simulink model "JSimResultsModel2"  (R2021a)
settings: Solver=VariableStepAuto  StartTime=0.0  StopTime=25  RelTol=1e-3
values from neighbouring files (symbols this model uses):
  A = obj.networkMatrices.A    [Network.m]    (also in Subsystem.m = obj.A{obj.index}; jPaperData1.mat = [7.21225729966 1.39049686205 0 0 -0.282509513675 -0.19440187; jPaperData2.mat = [1.59283418225 -1.98990334273 -0.0774022354425 0.03883188575; paperData.mat = [-0.897343897753 -1.03363634124 0 0 0 0 -1.03363634124 -1.19)
  AcDiss =     [jPaperData1.mat]    (also in jPaperData2.mat)
  AcStab =     [jPaperData1.mat]    (also in jPaperData2.mat = [-4.66639923531 0.0224905641012 0.183856829633 -0.0600919958)
  B = obj.networkMatrices.B    [Network.m]    (also in Subsystem.m = obj.B{obj.index}; jPaperData1.mat = [0.133289291835 -2.25582289472 0 0 0 0 0 0 0 0 0 0 ... (50 e; jPaperData2.mat = [0.884783010265 -0.0578061269532 0 0 0 0 0 0 0 0 0 0 ... (50; paperData.mat = [-0.767652209467 0.0479827696564 0 0 0 0 0 0 0 0.69770450426)
  BcDiss =     [jPaperData1.mat]    (also in jPaperData2.mat)
  BcStab =     [jPaperData1.mat]    (also in jPaperData2.mat = [4.69331758427 -3.97574466957 -0.18243601768 0.0596281142245)
  C = obj.networkMatrices.C    [Network.m]    (also in Subsystem.m = {}; jPaperData1.mat = [-0.398868811937 0 0 0 0 0.199769403633 0 0 0 0 0 0 ... (50 ; jPaperData2.mat = [-2.29277321488 0 0 0 0 1.99520966434 0 0 0 0 0 0.4731154890; paperData.mat = [-0.192732954692 0 0 0.794595441386 0 0 0 1.44304729411 0 0 )
  CcDiss =     [jPaperData1.mat]    (also in jPaperData2.mat)
  CcStab =     [jPaperData1.mat]    (also in jPaperData2.mat = [3.40584102634 0.0670370876354 0 -0.466213574125 0.023320064)
  D = obj.networkMatrices.D    [Network.m]    (also in Subsystem.m = {}; jPaperData1.mat = [0 0 0 0 0 0 0 0 0 0 0 0 ... (25 elements, 5x5)]; jPaperData2.mat = [0 0 0 0 0 0 0 0 0 0 0 0 ... (25 elements, 5x5)]; paperData.mat = [0  0  0; 0  0  0; 0  0  0])
  DcDiss =     [jPaperData1.mat]    (also in jPaperData2.mat)
  DcStab =     [jPaperData1.mat]    (also in jPaperData2.mat = [-0.559949680356 -0.0227155093389 0 0.0369895329508 0.048553)
  E = obj.networkMatrices.E    [Network.m]    (also in Subsystem.m = {}; jPaperData1.mat = [0.013736298283 0.0126277412194 0 0 0 -0.00335268402912 0 0.; jPaperData2.mat = [-0.000849733283809 -0.00431479261265 0.00356522747973 0.001; paperData.mat = [0 0.622727541957 0 0 0 0 -0.10315996141 -0.125734072536 0 -)
  F = obj.networkMatrices.F    [Network.m]    (also in Subsystem.m = {}; jPaperData1.mat = [0 0 0 0 0 0 0.00667542601126 0 0 0 0 0 ... (25 elements, 5x; jPaperData2.mat = [0 0 0 0 0 0 0 0 0 0 0 0 ... (25 elements, 5x5)]; paperData.mat = [0.160906008337  0  0; 0  0.0149076612258  0; 0  0  0])
  G = obj.networkMatrices.G    [Network.m]    (also in Subsystem.m = {}; jPaperData1.mat = [1 0 0 0 0 1 0 0 0 0 0 1 ... (50 elements, 5x10)]; jPaperData2.mat = [1 0 0 0 0 1 0 0 0 0 0 1 ... (50 elements, 5x10)])
  H = obj.networkMatrices.H    [Network.m]    (also in Subsystem.m = {}; jPaperData1.mat = [1 0 0 0 0 0 1 0 0 0 0 0 ... (25 elements, 5x5)]; jPaperData2.mat = [1 0 0 0 0 0 1 0 0 0 0 0 ... (25 elements, 5x5)])
  J = obj.networkMatrices.J    [Network.m]    (also in Subsystem.m = {}; jPaperData1.mat = [1 0 0 0 0 0 1 0 0 0 0 0 ... (25 elements, 5x5)]; jPaperData2.mat = [1 0 0 0 0 0 1 0 0 0 0 0 ... (25 elements, 5x5)])
  KDiss = [0 0 0 0 0 0 0 0 0 0 0 0 ... (50 elements, 5x10)]    [jPaperData1.mat]    (also in jPaperData2.mat)
  KStab =     [jPaperData1.mat]    (also in jPaperData2.mat = [-4.86369493868 -0.00198336219621 0 -0.960462012264 -0.04588)
  LDiss =     [jPaperData1.mat]    (also in jPaperData2.mat = [-3.49678545473 -0.771253400681 0.0276218519768 -0.070221237)
  LStab =     [jPaperData1.mat]    (also in jPaperData2.mat = [-2.23296914639 -0.236331029549 0.0275982481338 -0.070133150)
  n = size(A,1)    [Network.m]    (also in Subsystem.m = obj.dim_n; jPaperData1.mat = 10; jPaperData2.mat = 10; temp1.m)
undefined symbols (not defined in the file or in its folder): AcDissD, AcStabD, BcDissD, BcStabD, CcDissD, CcStabD, DcDissD, DcStabD, KDissD, KStabD, LDissD, LStabD
libraries: simulink x1
settings Model: Creator=Shirantha Welikala  LastModifiedBy=Shirantha Welikala

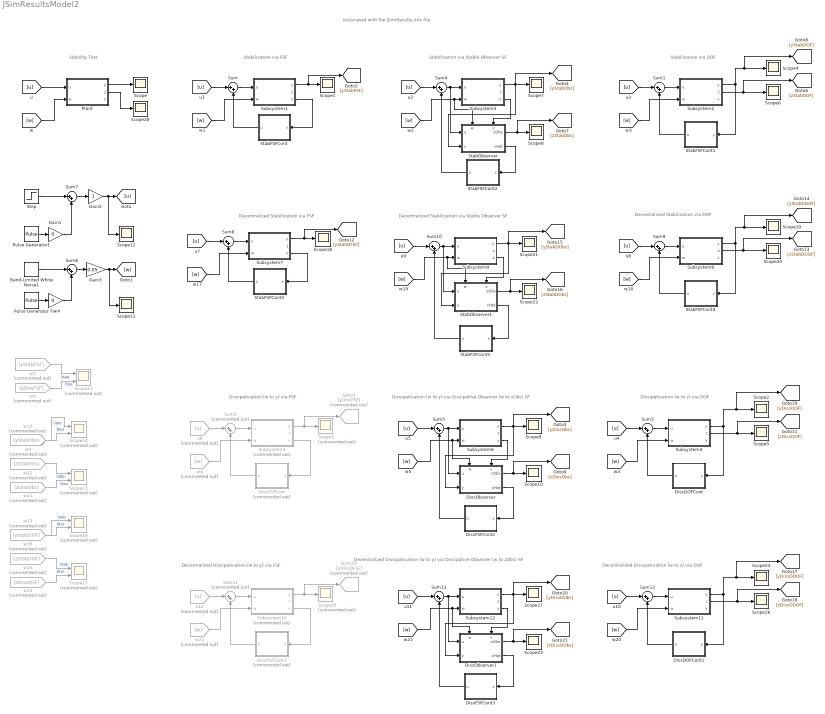
== system JSimResultsModel2 ==
  note: Associated with the JSimResults.mlx file
  note: Stability Test
  note: Stabilization via FSF
  note: Stabilization via DOF
  note: Dissipativation (w to y) via FSF
  note: Dissipativation (w to z) via DOF
  note: Stabilization via Stable Observer SF
  note: Dissipativation (w to y) via Dissipative Observer (w to zObs) SF
  note: Decentralized Stabilization via DOF
  note: Decentralized Stabilization via FSF
  note: Decentralized Stabilization via Stable Observer SF
  note: Decentralized Dissipativation (w to y) via FSF
  note: Decentralized Dissipativation (w to z) via DOF
  note: Decentralized Dissipativation (w to y) via Dissipative Observer (w to zObs) SF
  Band-Limited White Noise1 : simulink/Sources/Band-Limited White Noise  Cov=[1]  Ts=0.01  seed=[1;2;3;4;5]
  DissDOFCont : Subsystem
  DissDOFCont1 : Subsystem
  DissFSFCont : Subsystem  Commented=on
  DissFSFCont1 : Subsystem  Commented=on
  DissFSFCont2 : Subsystem
  DissFSFCont3 : Subsystem
  DissObserver : Subsystem
      settings: PortSchema="{\"entries\":[{\"content\":{\"sides\":[{\"content\":{\"connectorIds\":[\"In1\",\"In2\"]},\"type\":\"ConnectorPlacement.EquallySpacedRectSide\",\"uuid\":\"bb89ae44-d021-4487-97ea-d884edbfbdc6\"},{\"content\":{\"connectorIds\":[\"Out1\",\"Out2\"],\"side\":\"RIGHT\"},\"type\":\"ConnectorPlacement.EquallySpacedRectSide\",\"uuid\":\"8b439939-30ad-482f-a8e7-d460793e5232\"},{\"content\":{\"connectorIds\":[\"In3\",\"In4\"],\"side\":\"TOP\"},\"type\":\"ConnectorPlacement.EquallySpacedRectSide\",\"uuid\":\"831faa58-2099-4155-89c8-01b636ce25d5\"}]},\"type\":\"ConnectorPlacement.EquallySpacedConnector\",\"uuid\":\"0a775592-9d3b-4995-aaad-fe94d15f27f2\"}],\"packageUris\":[\"http://schema.mathworks.com/mf0/Connector/R2020b\"],\"version\":\"1.0\"}"
  DissObserver1 : Subsystem
      settings: PortSchema="{\"entries\":[{\"content\":{\"sides\":[{\"content\":{\"connectorIds\":[\"In1\",\"In2\"]},\"type\":\"ConnectorPlacement.EquallySpacedRectSide\",\"uuid\":\"bb89ae44-d021-4487-97ea-d884edbfbdc6\"},{\"content\":{\"connectorIds\":[\"Out1\",\"Out2\"],\"side\":\"RIGHT\"},\"type\":\"ConnectorPlacement.EquallySpacedRectSide\",\"uuid\":\"8b439939-30ad-482f-a8e7-d460793e5232\"},{\"content\":{\"connectorIds\":[\"In3\",\"In4\"],\"side\":\"TOP\"},\"type\":\"ConnectorPlacement.EquallySpacedRectSide\",\"uuid\":\"831faa58-2099-4155-89c8-01b636ce25d5\"}]},\"type\":\"ConnectorPlacement.EquallySpacedConnector\",\"uuid\":\"0a775592-9d3b-4995-aaad-fe94d15f27f2\"}],\"packageUris\":[\"http://schema.mathworks.com/mf0/Connector/R2020b\"],\"version\":\"1.0\"}"
  Gain : Gain  Gain=0
  Gain1 : Gain  Gain=0
  Gain2 : Gain
  Gain3 : Gain  Gain=0.05
  Goto19 : Goto  Commented=on  GotoTag=yDissDFSF
  Goto3 : Goto  Commented=on  GotoTag=yDissFSF
  Plant : Subsystem
  Pulse Generator : DiscretePulseGenerator  PulseType=Time based  Period=30  PulseWidth=10  PhaseDelay=[20;21;22;23;24]
  Pulse Generator1 : DiscretePulseGenerator  PulseType=Time based  Amplitude=0.5  Period=100  PulseWidth=5  PhaseDelay=[45;46;47;48;49]
  Scope{,1..2,4..12,18..24,26..28} (22 alike) : Scope
  Scope{13..17} (5 alike) : Scope  Commented=on  NumInputPorts=2
  Scope25 : Scope  Commented=on
  Scope3 : Scope  Commented=on
  StabFSFCont : Subsystem
  StabFSFCont1 : Subsystem
  StabFSFCont2 : Subsystem
  StabFSFCont3 : Subsystem
  StabFSFCont4 : Subsystem
  StabFSFCont5 : Subsystem
  StabObserver : Subsystem
      settings: PortSchema="{\"entries\":[{\"content\":{\"sides\":[{\"content\":{\"connectorIds\":[\"In1\",\"In2\"]},\"type\":\"ConnectorPlacement.EquallySpacedRectSide\",\"uuid\":\"bb89ae44-d021-4487-97ea-d884edbfbdc6\"},{\"content\":{\"connectorIds\":[\"Out1\",\"Out2\"],\"side\":\"RIGHT\"},\"type\":\"ConnectorPlacement.EquallySpacedRectSide\",\"uuid\":\"8b439939-30ad-482f-a8e7-d460793e5232\"},{\"content\":{\"connectorIds\":[\"In3\",\"In4\"],\"side\":\"TOP\"},\"type\":\"ConnectorPlacement.EquallySpacedRectSide\",\"uuid\":\"831faa58-2099-4155-89c8-01b636ce25d5\"}]},\"type\":\"ConnectorPlacement.EquallySpacedConnector\",\"uuid\":\"0a775592-9d3b-4995-aaad-fe94d15f27f2\"}],\"packageUris\":[\"http://schema.mathworks.com/mf0/Connector/R2020b\"],\"version\":\"1.0\"}"
  StabObserver1 : Subsystem
      settings: PortSchema="{\"entries\":[{\"content\":{\"sides\":[{\"content\":{\"connectorIds\":[\"In1\",\"In2\"]},\"type\":\"ConnectorPlacement.EquallySpacedRectSide\",\"uuid\":\"bb89ae44-d021-4487-97ea-d884edbfbdc6\"},{\"content\":{\"connectorIds\":[\"Out1\",\"Out2\"],\"side\":\"RIGHT\"},\"type\":\"ConnectorPlacement.EquallySpacedRectSide\",\"uuid\":\"8b439939-30ad-482f-a8e7-d460793e5232\"},{\"content\":{\"connectorIds\":[\"In3\",\"In4\"],\"side\":\"TOP\"},\"type\":\"ConnectorPlacement.EquallySpacedRectSide\",\"uuid\":\"831faa58-2099-4155-89c8-01b636ce25d5\"}]},\"type\":\"ConnectorPlacement.EquallySpacedConnector\",\"uuid\":\"0a775592-9d3b-4995-aaad-fe94d15f27f2\"}],\"packageUris\":[\"http://schema.mathworks.com/mf0/Connector/R2020b\"],\"version\":\"1.0\"}"
  Step : Step  Time=[5;6;7;8;9]  Before=1  After=0  SampleTime=0
  Subsystem1 : Subsystem
  Subsystem10 : Subsystem  Commented=on
  Subsystem11 : Subsystem
  Subsystem12 : Subsystem
  Subsystem2 : Subsystem
  Subsystem3 : Subsystem  Commented=on
  Subsystem4 : Subsystem
  Subsystem5 : Subsystem
  Subsystem6 : Subsystem
  Subsystem7 : Subsystem
  Subsystem8 : Subsystem
  Subsystem9 : Subsystem
  Sum{,1,3..10,12..13} (12 alike) : Sum  Inputs=|++
  Sum11 : Sum  Commented=on  Inputs=|++
  Sum2 : Sum  Commented=on  Inputs=|++
  u12 : From  Commented=on  GotoTag=u
  u6 : From  Commented=on  GotoTag=u
  w10 : From  Commented=on  GotoTag=yDissObs
  w11 : From  Commented=on  GotoTag=zDissObs
  w12 : From  Commented=on  GotoTag=zStabObs
  w13 : From  Commented=on  GotoTag=yDissDOF
  w14 : From  Commented=on  GotoTag=zDissDOF
  w15 : From  Commented=on  GotoTag=zStabDOF
  w16 : From  Commented=on  GotoTag=yStabDOF
  w22 : From  Commented=on  GotoTag=w
  w6 : From  Commented=on  GotoTag=w
  w7 : From  Commented=on  GotoTag=yStabFSF
  w8 : From  Commented=on  GotoTag=yDissFSF
  w9 : From  Commented=on  GotoTag=yStabObs
  wires:
  Plant/1(y) -> Scope/1
  [u] -> Plant/1(u)
  Subsystem1/1(y) -> [yStabFSF], Scope1/1
  Subsystem1/3(x) -> StabFSFCont/1(x)
  [u] -> Sum/1
  Sum/1 -> Subsystem1/1(u)
  StabFSFCont1/1(u) -> Sum1/2
  Subsystem2/1(y) -> [yStabDOF], Scope4/1, StabFSFCont1/1(y)
  Sum1/1 -> Subsystem2/1(u)
  [w] -> Subsystem1/2(w)
  [w] -> Plant/2(w)
  StabFSFCont/1(u) -> Sum/2
  Subsystem3/1(y) -> Goto3/1, Scope3/1
  Subsystem3/3(x) -> DissFSFCont/1(x)
  u6/1 -> Sum2/1
  Sum2/1 -> Subsystem3/1(u)
  DissFSFCont/1(u) -> Sum2/2
  Sum3/1 -> Subsystem4/1(u)
  [u] -> Sum3/1
  DissDOFCont/1(u) -> Sum3/2
  Subsystem4/1(y) -> DissDOFCont/1(y), Scope2/1, [yDissDOF]
  Subsystem4/2(z) -> [zDissDOF], Scope5/1
  Subsystem2/2(z) -> [zStabDOF], Scope6/1
  Sum4/1 -> StabObserver/1(u), Subsystem5/1(u)
  StabFSFCont2/1(u) -> Sum4/2
  Subsystem5/3(x) -> StabObserver/4(x)
  Subsystem5/1(y) -> Scope7/1, [yStabObs], StabObserver/2(y)
  StabObserver/1(zObs) -> [zStabObs], Scope8/1
  StabObserver/2(xHat) -> StabFSFCont2/1(x)
  DissObserver/2(xHat) -> DissFSFCont2/1(x)
  DissObserver/1(zObs) -> [zDissObs], Scope10/1
  Subsystem6/3(x) -> DissObserver/4(x)
  Sum5/1 -> DissObserver/1(u), Subsystem6/1(u)
  DissFSFCont2/1(u) -> Sum5/2
  Subsystem6/1(y) -> [yDissObs], DissObserver/2(y), Scope9/1
  [w] -> DissObserver/3(w), Subsystem6/2(w)
  Band-Limited White Noise1/1 -> Sum6/1
  Sum6/1 -> Gain3/1
  Gain/1 -> Sum6/2
  Pulse Generator/1 -> Gain/1
  Gain1/1 -> Sum7/2
  Sum7/1 -> Gain2/1
  Pulse Generator1/1 -> Gain1/1
  Step/1 -> Sum7/1
  [u] -> Sum4/1
  [w] -> StabObserver/3(w), Subsystem5/2(w)
  w6/1 -> Subsystem3/2(w)
  [u] -> Sum5/1
  [w] -> Subsystem4/2(w)
  [u] -> Sum1/1
  [w] -> Subsystem2/2(w)
  w7/1 -> Scope13/1  "Stab"
  w8/1 -> Scope13/2  "Diss"
  w10/1 -> Scope14/2  "Diss"
  w9/1 -> Scope14/1  "Stab"
  w12/1 -> Scope15/1  "Stab"
  w11/1 -> Scope15/2  "Diss"
  w16/1 -> Scope16/1  "Stab"
  w14/1 -> Scope17/2  "Diss"
  w15/1 -> Scope17/1  "Stab"
  w13/1 -> Scope16/2  "Diss"
  Gain2/1 -> Scope12/1, [u]
  Sum8/1 -> Subsystem7/1(u)
  [u] -> Sum8/1
  StabFSFCont3/1(u) -> Sum8/2
  Subsystem7/3(x) -> StabFSFCont3/1(x)
  [w] -> Subsystem7/2(w)
  Subsystem7/1(y) -> [yStabDFSF], Scope18/1
  Gain3/1 -> Scope11/1, [w]
  [u] -> Sum9/1
  [w] -> Subsystem8/2(w)
  StabFSFCont4/1(u) -> Sum9/2
  Subsystem8/1(y) -> [yStabDDOF], Scope19/1, StabFSFCont4/1(y)
  Sum9/1 -> Subsystem8/1(u)
  Subsystem8/2(z) -> [zStabDDOF], Scope20/1
  Subsystem9/1(y) -> Scope21/1, [yStabDObs], StabObserver1/2(y)
  [w] -> StabObserver1/3(w), Subsystem9/2(w)
  Subsystem9/3(x) -> StabObserver1/4(x)
  StabObserver1/1(zObs) -> [zStabDObs], Scope22/1
  StabObserver1/2(xHat) -> StabFSFCont5/1(x)
  Sum10/1 -> StabObserver1/1(u), Subsystem9/1(u)
  [u] -> Sum10/1
  StabFSFCont5/1(u) -> Sum10/2
  [w] -> Subsystem11/2(w)
  [u] -> Sum13/1
  w22/1 -> Subsystem10/2(w)
  [w] -> Subsystem12/2(w), DissObserver1/3(w)
  Subsystem12/1(y) -> Scope27/1, DissObserver1/2(y), [yDissDObs]
  DissFSFCont3/1(u) -> Sum13/2
  Sum13/1 -> Subsystem12/1(u), DissObserver1/1(u)
  Subsystem12/3(x) -> DissObserver1/4(x)
  DissObserver1/1(zObs) -> Scope23/1, [zDissDObs]
  DissObserver1/2(xHat) -> DissFSFCont3/1(x)
  Subsystem11/2(z) -> Scope26/1, [zDissDDOF]
  Subsystem11/1(y) -> [yDissDDOF], Scope24/1, DissDOFCont1/1(y)
  DissDOFCont1/1(u) -> Sum12/2
  [u] -> Sum12/1
  Sum12/1 -> Subsystem11/1(u)
  DissFSFCont1/1(u) -> Sum11/2
  Sum11/1 -> Subsystem10/1(u)
  u12/1 -> Sum11/1
  Subsystem10/3(x) -> DissFSFCont1/1(x)
  Subsystem10/1(y) -> Scope25/1, Goto19/1
  Plant/2(z) -> Scope28/1

== system JSimResultsModel2/DissDOFCont ==
  y : Inport
  State-Space : StateSpace  A=AcDiss  B=BcDiss  C=CcDiss  D=DcDiss  InitialCondition=zeros(n,1)
  u : Outport
  wires:
  y/1 -> State-Space/1
  State-Space/1 -> u/1

== system JSimResultsModel2/DissDOFCont1 ==
  y : Inport
  State-Space : StateSpace  A=AcDissD  B=BcDissD  C=CcDissD  D=DcDissD  InitialCondition=zeros(n,1)
  u : Outport
  wires:
  State-Space/1 -> u/1
  y/1 -> State-Space/1

== system JSimResultsModel2/DissFSFCont ==
  x : Inport
  Gain : Gain  Gain=KDiss  Multiplication=Matrix(K*u)
  u : Outport
  wires:
  x/1 -> Gain/1
  Gain/1 -> u/1

== system JSimResultsModel2/DissFSFCont1 ==
  x : Inport
  Gain : Gain  Gain=KDissD  Multiplication=Matrix(K*u)
  u : Outport
  wires:
  Gain/1 -> u/1
  x/1 -> Gain/1

== system JSimResultsModel2/DissFSFCont2 ==
  x : Inport
  Gain : Gain  Gain=KStab  Multiplication=Matrix(K*u)
  u : Outport
  wires:
  x/1 -> Gain/1
  Gain/1 -> u/1

== system JSimResultsModel2/DissFSFCont3 ==
  x : Inport
  Gain : Gain  Gain=KStabD  Multiplication=Matrix(K*u)
  u : Outport
  wires:
  Gain/1 -> u/1
  x/1 -> Gain/1

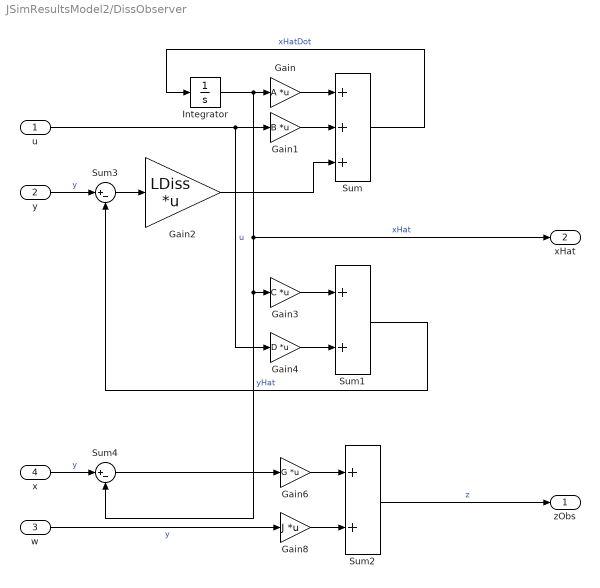
== system JSimResultsModel2/DissObserver ==
  u : Inport
  y : Inport  Port=2
  w : Inport  Port=3
  x : Inport  Port=4
  Gain : Gain  Gain=A  Multiplication=Matrix(K*u)
  Gain1 : Gain  Gain=B  Multiplication=Matrix(K*u)
  Gain2 : Gain  Gain=LDiss  Multiplication=Matrix(K*u)
  Gain3 : Gain  Gain=C  Multiplication=Matrix(K*u)
  Gain4 : Gain  Gain=D  Multiplication=Matrix(K*u)
  Gain6 : Gain  Gain=G  Multiplication=Matrix(K*u)
  Gain8 : Gain  Gain=J  Multiplication=Matrix(K*u)
  Integrator : Integrator  InitialCondition=zeros(n,1)
  Sum : Sum  Inputs=+++
  Sum1 : Sum
  Sum2 : Sum
  Sum3 : Sum  Inputs=|+-
  Sum4 : Sum  Inputs=|+-
  zObs : Outport
  xHat : Outport  Port=2
  wires:
  Gain2/1 -> Sum/3
  Sum/1 -> Integrator/1  "xHatDot"
  Gain/1 -> Sum/1
  Gain1/1 -> Sum/2
  Integrator/1 -> Sum4/2, Gain3/1, xHat/1, Gain/1  "xHat"
  Sum2/1 -> zObs/1  "z"
  Gain8/1 -> Sum2/2
  Gain6/1 -> Sum2/1
  u/1 -> Gain1/1, Gain4/1  "u"
  Gain4/1 -> Sum1/2
  Sum1/1 -> Sum3/2  "yHat"
  Gain3/1 -> Sum1/1
  y/1 -> Sum3/1  "y"
  Sum3/1 -> Gain2/1
  x/1 -> Sum4/1  "y"
  Sum4/1 -> Gain6/1
  w/1 -> Gain8/1  "y"

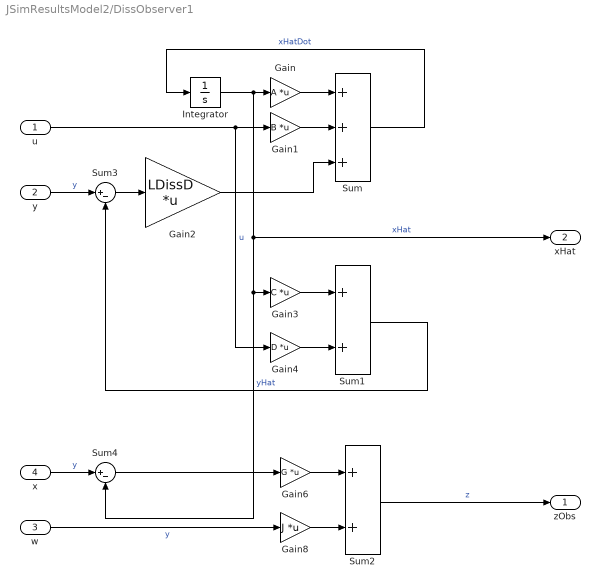
== system JSimResultsModel2/DissObserver1 ==
  u : Inport
  y : Inport  Port=2
  w : Inport  Port=3
  x : Inport  Port=4
  Gain : Gain  Gain=A  Multiplication=Matrix(K*u)
  Gain1 : Gain  Gain=B  Multiplication=Matrix(K*u)
  Gain2 : Gain  Gain=LDissD  Multiplication=Matrix(K*u)
  Gain3 : Gain  Gain=C  Multiplication=Matrix(K*u)
  Gain4 : Gain  Gain=D  Multiplication=Matrix(K*u)
  Gain6 : Gain  Gain=G  Multiplication=Matrix(K*u)
  Gain8 : Gain  Gain=J  Multiplication=Matrix(K*u)
  Integrator : Integrator  InitialCondition=zeros(n,1)
  Sum : Sum  Inputs=+++
  Sum1 : Sum
  Sum2 : Sum
  Sum3 : Sum  Inputs=|+-
  Sum4 : Sum  Inputs=|+-
  zObs : Outport
  xHat : Outport  Port=2
  wires:
  w/1 -> Gain8/1  "y"
  Sum4/1 -> Gain6/1
  x/1 -> Sum4/1  "y"
  Sum3/1 -> Gain2/1
  y/1 -> Sum3/1  "y"
  Gain3/1 -> Sum1/1
  Sum1/1 -> Sum3/2  "yHat"
  Gain4/1 -> Sum1/2
  u/1 -> Gain4/1, Gain1/1  "u"
  Gain6/1 -> Sum2/1
  Gain8/1 -> Sum2/2
  Sum2/1 -> zObs/1  "z"
  Integrator/1 -> Gain/1, xHat/1, Gain3/1, Sum4/2  "xHat"
  Gain1/1 -> Sum/2
  Gain/1 -> Sum/1
  Sum/1 -> Integrator/1  "xHatDot"
  Gain2/1 -> Sum/3

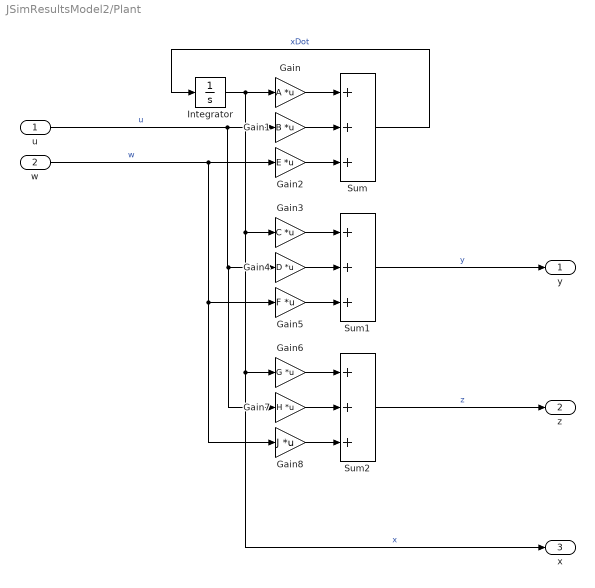
== system JSimResultsModel2/Plant ==
  u : Inport
  w : Inport  Port=2
  Gain : Gain  Gain=A  Multiplication=Matrix(K*u)
  Gain1 : Gain  Gain=B  Multiplication=Matrix(K*u)
  Gain2 : Gain  Gain=E  Multiplication=Matrix(K*u)
  Gain3 : Gain  Gain=C  Multiplication=Matrix(K*u)
  Gain4 : Gain  Gain=D  Multiplication=Matrix(K*u)
  Gain5 : Gain  Gain=F  Multiplication=Matrix(K*u)
  Gain6 : Gain  Gain=G  Multiplication=Matrix(K*u)
  Gain7 : Gain  Gain=H  Multiplication=Matrix(K*u)
  Gain8 : Gain  Gain=J  Multiplication=Matrix(K*u)
  Integrator : Integrator  InitialCondition=10*ones(n,1)
  Sum : Sum  Inputs=+++
  Sum1 : Sum  Inputs=+++
  Sum2 : Sum  Inputs=+++
  y : Outport
  z : Outport  Port=2
  x : Outport  Port=3
  wires:
  u/1 -> Gain7/1, Gain4/1, Gain1/1  "u"
  Gain2/1 -> Sum/3
  w/1 -> Gain8/1, Gain5/1, Gain2/1  "w"
  Gain3/1 -> Sum1/1
  Sum/1 -> Integrator/1  "xDot"
  Gain5/1 -> Sum1/3
  Gain/1 -> Sum/1
  Gain1/1 -> Sum/2
  Gain4/1 -> Sum1/2
  Sum2/1 -> z/1  "z"
  Sum1/1 -> y/1  "y"
  Gain8/1 -> Sum2/3
  Gain6/1 -> Sum2/1
  Gain7/1 -> Sum2/2
  Integrator/1 -> x/1, Gain6/1, Gain3/1, Gain/1  "x"

== system JSimResultsModel2/StabFSFCont ==
  x : Inport
  Gain : Gain  Gain=KStab  Multiplication=Matrix(K*u)
  u : Outport
  wires:
  x/1 -> Gain/1
  Gain/1 -> u/1

== system JSimResultsModel2/StabFSFCont1 ==
  y : Inport
  State-Space : StateSpace  A=AcStab  B=BcStab  C=CcStab  D=DcStab  InitialCondition=zeros(n,1)
  u : Outport
  wires:
  y/1 -> State-Space/1
  State-Space/1 -> u/1

== system JSimResultsModel2/StabFSFCont2 ==
  x : Inport
  Gain : Gain  Gain=KStab  Multiplication=Matrix(K*u)
  u : Outport
  wires:
  x/1 -> Gain/1
  Gain/1 -> u/1

== system JSimResultsModel2/StabFSFCont3 ==
  x : Inport
  Gain : Gain  Gain=KStabD  Multiplication=Matrix(K*u)
  u : Outport
  wires:
  x/1 -> Gain/1
  Gain/1 -> u/1

== system JSimResultsModel2/StabFSFCont4 ==
  y : Inport
  State-Space : StateSpace  A=AcStabD  B=BcStabD  C=CcStabD  D=DcStabD  InitialCondition=zeros(n,1)
  u : Outport
  wires:
  y/1 -> State-Space/1
  State-Space/1 -> u/1

== system JSimResultsModel2/StabFSFCont5 ==
  x : Inport
  Gain : Gain  Gain=KStabD  Multiplication=Matrix(K*u)
  u : Outport
  wires:
  x/1 -> Gain/1
  Gain/1 -> u/1

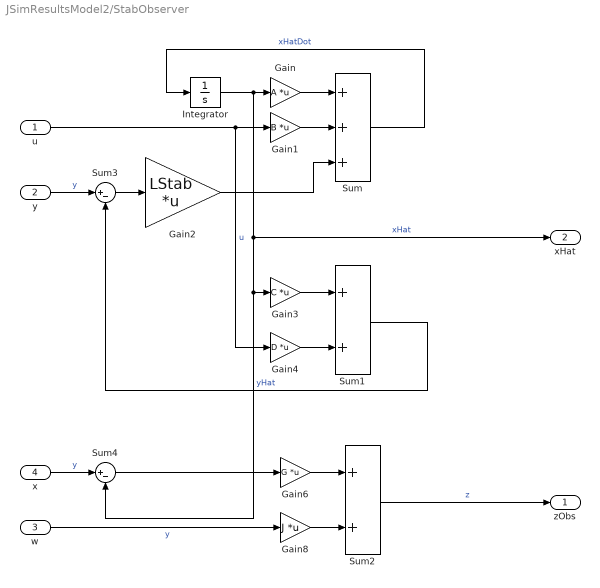
== system JSimResultsModel2/StabObserver ==
  u : Inport
  y : Inport  Port=2
  w : Inport  Port=3
  x : Inport  Port=4
  Gain : Gain  Gain=A  Multiplication=Matrix(K*u)
  Gain1 : Gain  Gain=B  Multiplication=Matrix(K*u)
  Gain2 : Gain  Gain=LStab  Multiplication=Matrix(K*u)
  Gain3 : Gain  Gain=C  Multiplication=Matrix(K*u)
  Gain4 : Gain  Gain=D  Multiplication=Matrix(K*u)
  Gain6 : Gain  Gain=G  Multiplication=Matrix(K*u)
  Gain8 : Gain  Gain=J  Multiplication=Matrix(K*u)
  Integrator : Integrator  InitialCondition=zeros(n,1)
  Sum : Sum  Inputs=+++
  Sum1 : Sum
  Sum2 : Sum
  Sum3 : Sum  Inputs=|+-
  Sum4 : Sum  Inputs=|+-
  zObs : Outport
  xHat : Outport  Port=2
  wires:
  Gain2/1 -> Sum/3
  Sum/1 -> Integrator/1  "xHatDot"
  Gain/1 -> Sum/1
  Gain1/1 -> Sum/2
  Integrator/1 -> Sum4/2, Gain3/1, xHat/1, Gain/1  "xHat"
  Sum2/1 -> zObs/1  "z"
  Gain8/1 -> Sum2/2
  Gain6/1 -> Sum2/1
  u/1 -> Gain1/1, Gain4/1  "u"
  Gain4/1 -> Sum1/2
  Sum1/1 -> Sum3/2  "yHat"
  Gain3/1 -> Sum1/1
  y/1 -> Sum3/1  "y"
  Sum3/1 -> Gain2/1
  x/1 -> Sum4/1  "y"
  Sum4/1 -> Gain6/1
  w/1 -> Gain8/1  "y"

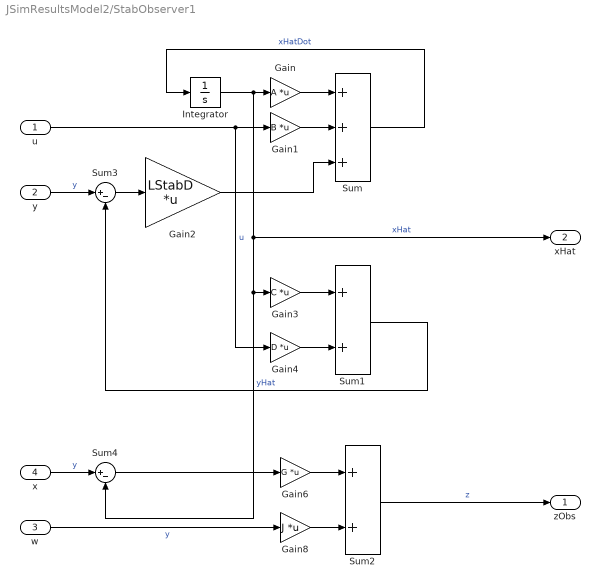
== system JSimResultsModel2/StabObserver1 ==
  u : Inport
  y : Inport  Port=2
  w : Inport  Port=3
  x : Inport  Port=4
  Gain : Gain  Gain=A  Multiplication=Matrix(K*u)
  Gain1 : Gain  Gain=B  Multiplication=Matrix(K*u)
  Gain2 : Gain  Gain=LStabD  Multiplication=Matrix(K*u)
  Gain3 : Gain  Gain=C  Multiplication=Matrix(K*u)
  Gain4 : Gain  Gain=D  Multiplication=Matrix(K*u)
  Gain6 : Gain  Gain=G  Multiplication=Matrix(K*u)
  Gain8 : Gain  Gain=J  Multiplication=Matrix(K*u)
  Integrator : Integrator  InitialCondition=zeros(n,1)
  Sum : Sum  Inputs=+++
  Sum1 : Sum
  Sum2 : Sum
  Sum3 : Sum  Inputs=|+-
  Sum4 : Sum  Inputs=|+-
  zObs : Outport
  xHat : Outport  Port=2
  wires:
  Gain2/1 -> Sum/3
  Sum/1 -> Integrator/1  "xHatDot"
  Gain/1 -> Sum/1
  Gain1/1 -> Sum/2
  Integrator/1 -> Sum4/2, Gain3/1, xHat/1, Gain/1  "xHat"
  Sum2/1 -> zObs/1  "z"
  Gain8/1 -> Sum2/2
  Gain6/1 -> Sum2/1
  u/1 -> Gain1/1, Gain4/1  "u"
  Gain4/1 -> Sum1/2
  Sum1/1 -> Sum3/2  "yHat"
  Gain3/1 -> Sum1/1
  y/1 -> Sum3/1  "y"
  Sum3/1 -> Gain2/1
  x/1 -> Sum4/1  "y"
  Sum4/1 -> Gain6/1
  w/1 -> Gain8/1  "y"

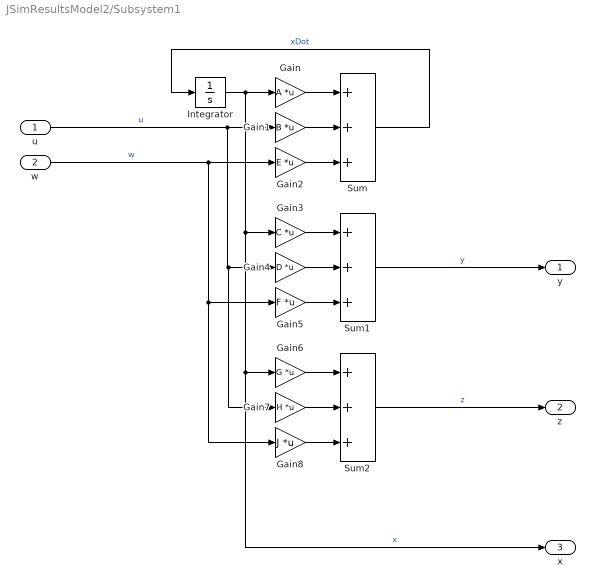
== system JSimResultsModel2/Subsystem1 ==
  u : Inport
  w : Inport  Port=2
  Gain : Gain  Gain=A  Multiplication=Matrix(K*u)
  Gain1 : Gain  Gain=B  Multiplication=Matrix(K*u)
  Gain2 : Gain  Gain=E  Multiplication=Matrix(K*u)
  Gain3 : Gain  Gain=C  Multiplication=Matrix(K*u)
  Gain4 : Gain  Gain=D  Multiplication=Matrix(K*u)
  Gain5 : Gain  Gain=F  Multiplication=Matrix(K*u)
  Gain6 : Gain  Gain=G  Multiplication=Matrix(K*u)
  Gain7 : Gain  Gain=H  Multiplication=Matrix(K*u)
  Gain8 : Gain  Gain=J  Multiplication=Matrix(K*u)
  Integrator : Integrator  InitialCondition=10*ones(n,1)
  Sum : Sum  Inputs=+++
  Sum1 : Sum  Inputs=+++
  Sum2 : Sum  Inputs=+++
  y : Outport
  z : Outport  Port=2
  x : Outport  Port=3
  wires:
  u/1 -> Gain7/1, Gain4/1, Gain1/1  "u"
  Gain2/1 -> Sum/3
  w/1 -> Gain8/1, Gain5/1, Gain2/1  "w"
  Gain3/1 -> Sum1/1
  Sum/1 -> Integrator/1  "xDot"
  Gain5/1 -> Sum1/3
  Gain/1 -> Sum/1
  Gain1/1 -> Sum/2
  Integrator/1 -> x/1, Gain6/1, Gain3/1, Gain/1  "x"
  Gain4/1 -> Sum1/2
  Sum2/1 -> z/1  "z"
  Sum1/1 -> y/1  "y"
  Gain8/1 -> Sum2/3
  Gain6/1 -> Sum2/1
  Gain7/1 -> Sum2/2

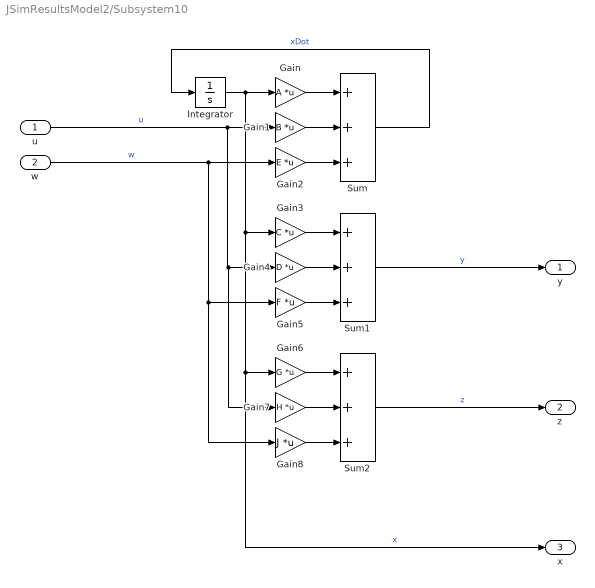
== system JSimResultsModel2/Subsystem10 ==
  u : Inport
  w : Inport  Port=2
  Gain : Gain  Gain=A  Multiplication=Matrix(K*u)
  Gain1 : Gain  Gain=B  Multiplication=Matrix(K*u)
  Gain2 : Gain  Gain=E  Multiplication=Matrix(K*u)
  Gain3 : Gain  Gain=C  Multiplication=Matrix(K*u)
  Gain4 : Gain  Gain=D  Multiplication=Matrix(K*u)
  Gain5 : Gain  Gain=F  Multiplication=Matrix(K*u)
  Gain6 : Gain  Gain=G  Multiplication=Matrix(K*u)
  Gain7 : Gain  Gain=H  Multiplication=Matrix(K*u)
  Gain8 : Gain  Gain=J  Multiplication=Matrix(K*u)
  Integrator : Integrator  InitialCondition=10*ones(n,1)
  Sum : Sum  Inputs=+++
  Sum1 : Sum  Inputs=+++
  Sum2 : Sum  Inputs=+++
  y : Outport
  z : Outport  Port=2
  x : Outport  Port=3
  wires:
  Gain7/1 -> Sum2/2
  Gain6/1 -> Sum2/1
  Gain8/1 -> Sum2/3
  Sum1/1 -> y/1  "y"
  Sum2/1 -> z/1  "z"
  Gain4/1 -> Sum1/2
  Integrator/1 -> Gain/1, Gain3/1, Gain6/1, x/1  "x"
  Gain1/1 -> Sum/2
  Gain/1 -> Sum/1
  Gain5/1 -> Sum1/3
  Sum/1 -> Integrator/1  "xDot"
  Gain3/1 -> Sum1/1
  w/1 -> Gain2/1, Gain5/1, Gain8/1  "w"
  Gain2/1 -> Sum/3
  u/1 -> Gain1/1, Gain4/1, Gain7/1  "u"

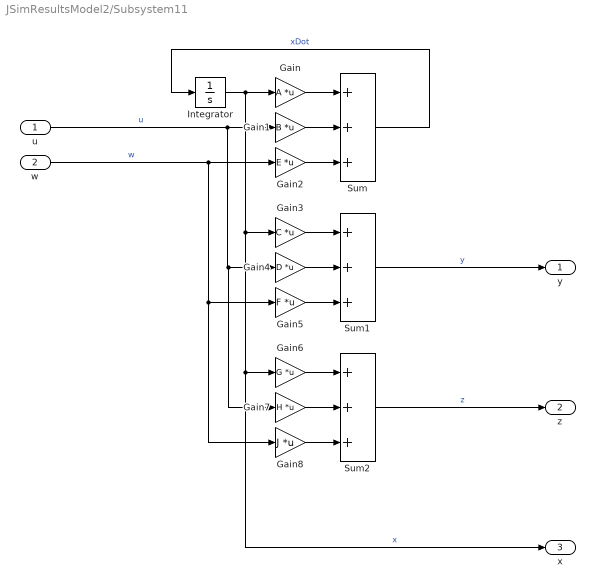
== system JSimResultsModel2/Subsystem11 ==
  u : Inport
  w : Inport  Port=2
  Gain : Gain  Gain=A  Multiplication=Matrix(K*u)
  Gain1 : Gain  Gain=B  Multiplication=Matrix(K*u)
  Gain2 : Gain  Gain=E  Multiplication=Matrix(K*u)
  Gain3 : Gain  Gain=C  Multiplication=Matrix(K*u)
  Gain4 : Gain  Gain=D  Multiplication=Matrix(K*u)
  Gain5 : Gain  Gain=F  Multiplication=Matrix(K*u)
  Gain6 : Gain  Gain=G  Multiplication=Matrix(K*u)
  Gain7 : Gain  Gain=H  Multiplication=Matrix(K*u)
  Gain8 : Gain  Gain=J  Multiplication=Matrix(K*u)
  Integrator : Integrator  InitialCondition=10*ones(n,1)
  Sum : Sum  Inputs=+++
  Sum1 : Sum  Inputs=+++
  Sum2 : Sum  Inputs=+++
  y : Outport
  z : Outport  Port=2
  x : Outport  Port=3
  wires:
  Gain7/1 -> Sum2/2
  Gain6/1 -> Sum2/1
  Gain8/1 -> Sum2/3
  Sum1/1 -> y/1  "y"
  Sum2/1 -> z/1  "z"
  Gain4/1 -> Sum1/2
  Integrator/1 -> Gain/1, Gain3/1, Gain6/1, x/1  "x"
  Gain1/1 -> Sum/2
  Gain/1 -> Sum/1
  Gain5/1 -> Sum1/3
  Sum/1 -> Integrator/1  "xDot"
  Gain3/1 -> Sum1/1
  w/1 -> Gain2/1, Gain5/1, Gain8/1  "w"
  Gain2/1 -> Sum/3
  u/1 -> Gain1/1, Gain4/1, Gain7/1  "u"

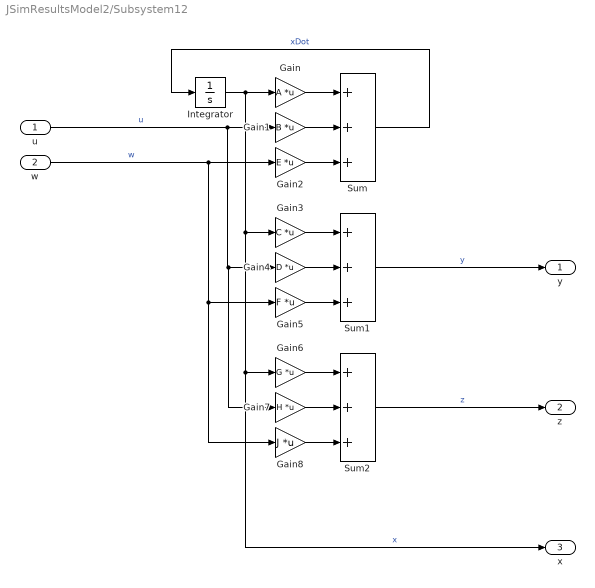
== system JSimResultsModel2/Subsystem12 ==
  u : Inport
  w : Inport  Port=2
  Gain : Gain  Gain=A  Multiplication=Matrix(K*u)
  Gain1 : Gain  Gain=B  Multiplication=Matrix(K*u)
  Gain2 : Gain  Gain=E  Multiplication=Matrix(K*u)
  Gain3 : Gain  Gain=C  Multiplication=Matrix(K*u)
  Gain4 : Gain  Gain=D  Multiplication=Matrix(K*u)
  Gain5 : Gain  Gain=F  Multiplication=Matrix(K*u)
  Gain6 : Gain  Gain=G  Multiplication=Matrix(K*u)
  Gain7 : Gain  Gain=H  Multiplication=Matrix(K*u)
  Gain8 : Gain  Gain=J  Multiplication=Matrix(K*u)
  Integrator : Integrator  InitialCondition=10*ones(n,1)
  Sum : Sum  Inputs=+++
  Sum1 : Sum  Inputs=+++
  Sum2 : Sum  Inputs=+++
  y : Outport
  z : Outport  Port=2
  x : Outport  Port=3
  wires:
  Gain7/1 -> Sum2/2
  Gain6/1 -> Sum2/1
  Gain8/1 -> Sum2/3
  Sum1/1 -> y/1  "y"
  Sum2/1 -> z/1  "z"
  Gain4/1 -> Sum1/2
  Integrator/1 -> Gain/1, Gain3/1, Gain6/1, x/1  "x"
  Gain1/1 -> Sum/2
  Gain/1 -> Sum/1
  Gain5/1 -> Sum1/3
  Sum/1 -> Integrator/1  "xDot"
  Gain3/1 -> Sum1/1
  w/1 -> Gain2/1, Gain5/1, Gain8/1  "w"
  Gain2/1 -> Sum/3
  u/1 -> Gain1/1, Gain4/1, Gain7/1  "u"

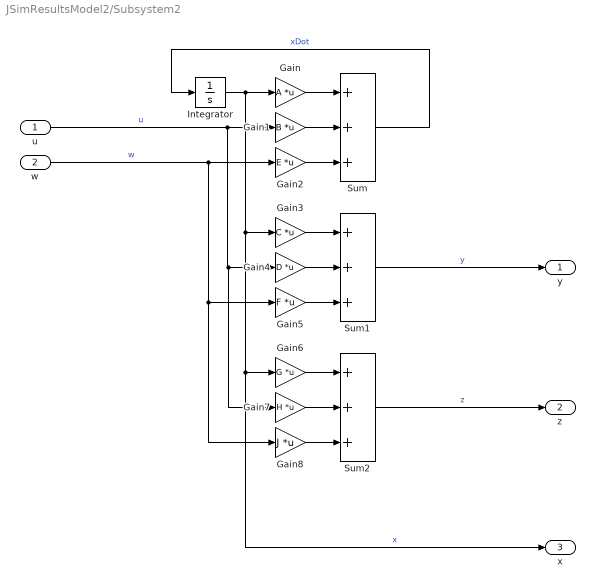
== system JSimResultsModel2/Subsystem2 ==
  u : Inport
  w : Inport  Port=2
  Gain : Gain  Gain=A  Multiplication=Matrix(K*u)
  Gain1 : Gain  Gain=B  Multiplication=Matrix(K*u)
  Gain2 : Gain  Gain=E  Multiplication=Matrix(K*u)
  Gain3 : Gain  Gain=C  Multiplication=Matrix(K*u)
  Gain4 : Gain  Gain=D  Multiplication=Matrix(K*u)
  Gain5 : Gain  Gain=F  Multiplication=Matrix(K*u)
  Gain6 : Gain  Gain=G  Multiplication=Matrix(K*u)
  Gain7 : Gain  Gain=H  Multiplication=Matrix(K*u)
  Gain8 : Gain  Gain=J  Multiplication=Matrix(K*u)
  Integrator : Integrator  InitialCondition=10*ones(n,1)
  Sum : Sum  Inputs=+++
  Sum1 : Sum  Inputs=+++
  Sum2 : Sum  Inputs=+++
  y : Outport
  z : Outport  Port=2
  x : Outport  Port=3
  wires:
  u/1 -> Gain7/1, Gain4/1, Gain1/1  "u"
  Gain2/1 -> Sum/3
  w/1 -> Gain8/1, Gain5/1, Gain2/1  "w"
  Gain3/1 -> Sum1/1
  Sum/1 -> Integrator/1  "xDot"
  Gain5/1 -> Sum1/3
  Gain/1 -> Sum/1
  Gain1/1 -> Sum/2
  Integrator/1 -> x/1, Gain6/1, Gain3/1, Gain/1  "x"
  Gain4/1 -> Sum1/2
  Sum2/1 -> z/1  "z"
  Sum1/1 -> y/1  "y"
  Gain8/1 -> Sum2/3
  Gain6/1 -> Sum2/1
  Gain7/1 -> Sum2/2

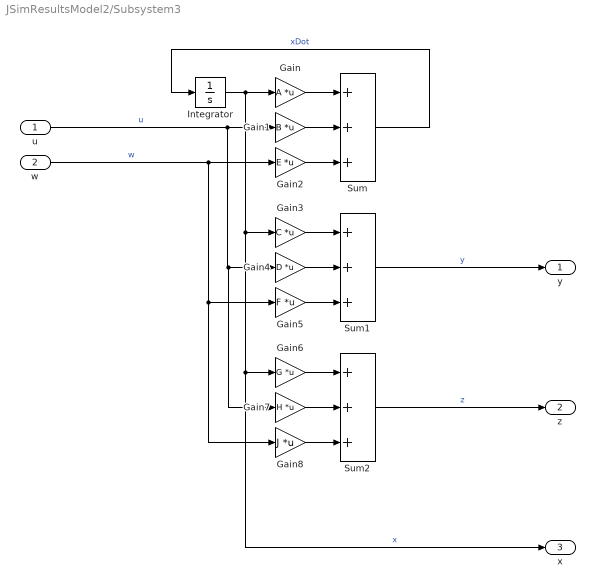
== system JSimResultsModel2/Subsystem3 ==
  u : Inport
  w : Inport  Port=2
  Gain : Gain  Gain=A  Multiplication=Matrix(K*u)
  Gain1 : Gain  Gain=B  Multiplication=Matrix(K*u)
  Gain2 : Gain  Gain=E  Multiplication=Matrix(K*u)
  Gain3 : Gain  Gain=C  Multiplication=Matrix(K*u)
  Gain4 : Gain  Gain=D  Multiplication=Matrix(K*u)
  Gain5 : Gain  Gain=F  Multiplication=Matrix(K*u)
  Gain6 : Gain  Gain=G  Multiplication=Matrix(K*u)
  Gain7 : Gain  Gain=H  Multiplication=Matrix(K*u)
  Gain8 : Gain  Gain=J  Multiplication=Matrix(K*u)
  Integrator : Integrator  InitialCondition=10*ones(n,1)
  Sum : Sum  Inputs=+++
  Sum1 : Sum  Inputs=+++
  Sum2 : Sum  Inputs=+++
  y : Outport
  z : Outport  Port=2
  x : Outport  Port=3
  wires:
  u/1 -> Gain7/1, Gain4/1, Gain1/1  "u"
  Gain2/1 -> Sum/3
  w/1 -> Gain8/1, Gain5/1, Gain2/1  "w"
  Gain3/1 -> Sum1/1
  Sum/1 -> Integrator/1  "xDot"
  Gain5/1 -> Sum1/3
  Gain/1 -> Sum/1
  Gain1/1 -> Sum/2
  Integrator/1 -> x/1, Gain6/1, Gain3/1, Gain/1  "x"
  Gain4/1 -> Sum1/2
  Sum2/1 -> z/1  "z"
  Sum1/1 -> y/1  "y"
  Gain8/1 -> Sum2/3
  Gain6/1 -> Sum2/1
  Gain7/1 -> Sum2/2

== system JSimResultsModel2/Subsystem4 ==
  u : Inport
  w : Inport  Port=2
  Gain : Gain  Gain=A  Multiplication=Matrix(K*u)
  Gain1 : Gain  Gain=B  Multiplication=Matrix(K*u)
  Gain2 : Gain  Gain=E  Multiplication=Matrix(K*u)
  Gain3 : Gain  Gain=C  Multiplication=Matrix(K*u)
  Gain4 : Gain  Gain=D  Multiplication=Matrix(K*u)
  Gain5 : Gain  Gain=F  Multiplication=Matrix(K*u)
  Gain6 : Gain  Gain=G  Multiplication=Matrix(K*u)
  Gain7 : Gain  Gain=H  Multiplication=Matrix(K*u)
  Gain8 : Gain  Gain=J  Multiplication=Matrix(K*u)
  Integrator : Integrator  InitialCondition=10*ones(n,1)
  Sum : Sum  Inputs=+++
  Sum1 : Sum  Inputs=+++
  Sum2 : Sum  Inputs=+++
  y : Outport
  z : Outport  Port=2
  x : Outport  Port=3
  wires:
  u/1 -> Gain7/1, Gain4/1, Gain1/1  "u"
  Gain2/1 -> Sum/3
  w/1 -> Gain8/1, Gain5/1, Gain2/1  "w"
  Gain3/1 -> Sum1/1
  Sum/1 -> Integrator/1  "xDot"
  Gain5/1 -> Sum1/3
  Gain/1 -> Sum/1
  Gain1/1 -> Sum/2
  Integrator/1 -> x/1, Gain6/1, Gain3/1, Gain/1  "x"
  Gain4/1 -> Sum1/2
  Sum2/1 -> z/1  "z"
  Sum1/1 -> y/1  "y"
  Gain8/1 -> Sum2/3
  Gain6/1 -> Sum2/1
  Gain7/1 -> Sum2/2

== system JSimResultsModel2/Subsystem5 ==
  u : Inport
  w : Inport  Port=2
  Gain : Gain  Gain=A  Multiplication=Matrix(K*u)
  Gain1 : Gain  Gain=B  Multiplication=Matrix(K*u)
  Gain2 : Gain  Gain=E  Multiplication=Matrix(K*u)
  Gain3 : Gain  Gain=C  Multiplication=Matrix(K*u)
  Gain4 : Gain  Gain=D  Multiplication=Matrix(K*u)
  Gain5 : Gain  Gain=F  Multiplication=Matrix(K*u)
  Gain6 : Gain  Gain=G  Multiplication=Matrix(K*u)
  Gain7 : Gain  Gain=H  Multiplication=Matrix(K*u)
  Gain8 : Gain  Gain=J  Multiplication=Matrix(K*u)
  Integrator : Integrator  InitialCondition=10*ones(n,1)
  Sum : Sum  Inputs=+++
  Sum1 : Sum  Inputs=+++
  Sum2 : Sum  Inputs=+++
  y : Outport
  z : Outport  Port=2
  x : Outport  Port=3
  wires:
  u/1 -> Gain7/1, Gain4/1, Gain1/1  "u"
  Gain2/1 -> Sum/3
  w/1 -> Gain8/1, Gain5/1, Gain2/1  "w"
  Gain3/1 -> Sum1/1
  Sum/1 -> Integrator/1  "xDot"
  Gain5/1 -> Sum1/3
  Gain/1 -> Sum/1
  Gain1/1 -> Sum/2
  Integrator/1 -> x/1, Gain6/1, Gain3/1, Gain/1  "x"
  Gain4/1 -> Sum1/2
  Sum2/1 -> z/1  "z"
  Sum1/1 -> y/1  "y"
  Gain8/1 -> Sum2/3
  Gain6/1 -> Sum2/1
  Gain7/1 -> Sum2/2

== system JSimResultsModel2/Subsystem6 ==
  u : Inport
  w : Inport  Port=2
  Gain : Gain  Gain=A  Multiplication=Matrix(K*u)
  Gain1 : Gain  Gain=B  Multiplication=Matrix(K*u)
  Gain2 : Gain  Gain=E  Multiplication=Matrix(K*u)
  Gain3 : Gain  Gain=C  Multiplication=Matrix(K*u)
  Gain4 : Gain  Gain=D  Multiplication=Matrix(K*u)
  Gain5 : Gain  Gain=F  Multiplication=Matrix(K*u)
  Gain6 : Gain  Gain=G  Multiplication=Matrix(K*u)
  Gain7 : Gain  Gain=H  Multiplication=Matrix(K*u)
  Gain8 : Gain  Gain=J  Multiplication=Matrix(K*u)
  Integrator : Integrator  InitialCondition=10*ones(n,1)
  Sum : Sum  Inputs=+++
  Sum1 : Sum  Inputs=+++
  Sum2 : Sum  Inputs=+++
  y : Outport
  z : Outport  Port=2
  x : Outport  Port=3
  wires:
  u/1 -> Gain7/1, Gain4/1, Gain1/1  "u"
  Gain2/1 -> Sum/3
  w/1 -> Gain8/1, Gain5/1, Gain2/1  "w"
  Gain3/1 -> Sum1/1
  Sum/1 -> Integrator/1  "xDot"
  Gain5/1 -> Sum1/3
  Gain/1 -> Sum/1
  Gain1/1 -> Sum/2
  Integrator/1 -> x/1, Gain6/1, Gain3/1, Gain/1  "x"
  Gain4/1 -> Sum1/2
  Sum2/1 -> z/1  "z"
  Sum1/1 -> y/1  "y"
  Gain8/1 -> Sum2/3
  Gain6/1 -> Sum2/1
  Gain7/1 -> Sum2/2

== system JSimResultsModel2/Subsystem7 ==
  u : Inport
  w : Inport  Port=2
  Gain : Gain  Gain=A  Multiplication=Matrix(K*u)
  Gain1 : Gain  Gain=B  Multiplication=Matrix(K*u)
  Gain2 : Gain  Gain=E  Multiplication=Matrix(K*u)
  Gain3 : Gain  Gain=C  Multiplication=Matrix(K*u)
  Gain4 : Gain  Gain=D  Multiplication=Matrix(K*u)
  Gain5 : Gain  Gain=F  Multiplication=Matrix(K*u)
  Gain6 : Gain  Gain=G  Multiplication=Matrix(K*u)
  Gain7 : Gain  Gain=H  Multiplication=Matrix(K*u)
  Gain8 : Gain  Gain=J  Multiplication=Matrix(K*u)
  Integrator : Integrator  InitialCondition=10*ones(n,1)
  Sum : Sum  Inputs=+++
  Sum1 : Sum  Inputs=+++
  Sum2 : Sum  Inputs=+++
  y : Outport
  z : Outport  Port=2
  x : Outport  Port=3
  wires:
  u/1 -> Gain7/1, Gain4/1, Gain1/1  "u"
  Gain2/1 -> Sum/3
  w/1 -> Gain8/1, Gain5/1, Gain2/1  "w"
  Gain3/1 -> Sum1/1
  Sum/1 -> Integrator/1  "xDot"
  Gain5/1 -> Sum1/3
  Gain/1 -> Sum/1
  Gain1/1 -> Sum/2
  Integrator/1 -> x/1, Gain6/1, Gain3/1, Gain/1  "x"
  Gain4/1 -> Sum1/2
  Sum2/1 -> z/1  "z"
  Sum1/1 -> y/1  "y"
  Gain8/1 -> Sum2/3
  Gain6/1 -> Sum2/1
  Gain7/1 -> Sum2/2

== system JSimResultsModel2/Subsystem8 ==
  u : Inport
  w : Inport  Port=2
  Gain : Gain  Gain=A  Multiplication=Matrix(K*u)
  Gain1 : Gain  Gain=B  Multiplication=Matrix(K*u)
  Gain2 : Gain  Gain=E  Multiplication=Matrix(K*u)
  Gain3 : Gain  Gain=C  Multiplication=Matrix(K*u)
  Gain4 : Gain  Gain=D  Multiplication=Matrix(K*u)
  Gain5 : Gain  Gain=F  Multiplication=Matrix(K*u)
  Gain6 : Gain  Gain=G  Multiplication=Matrix(K*u)
  Gain7 : Gain  Gain=H  Multiplication=Matrix(K*u)
  Gain8 : Gain  Gain=J  Multiplication=Matrix(K*u)
  Integrator : Integrator  InitialCondition=10*ones(n,1)
  Sum : Sum  Inputs=+++
  Sum1 : Sum  Inputs=+++
  Sum2 : Sum  Inputs=+++
  y : Outport
  z : Outport  Port=2
  x : Outport  Port=3
  wires:
  u/1 -> Gain7/1, Gain4/1, Gain1/1  "u"
  Gain2/1 -> Sum/3
  w/1 -> Gain8/1, Gain5/1, Gain2/1  "w"
  Gain3/1 -> Sum1/1
  Sum/1 -> Integrator/1  "xDot"
  Gain5/1 -> Sum1/3
  Gain/1 -> Sum/1
  Gain1/1 -> Sum/2
  Integrator/1 -> x/1, Gain6/1, Gain3/1, Gain/1  "x"
  Gain4/1 -> Sum1/2
  Sum2/1 -> z/1  "z"
  Sum1/1 -> y/1  "y"
  Gain8/1 -> Sum2/3
  Gain6/1 -> Sum2/1
  Gain7/1 -> Sum2/2

== system JSimResultsModel2/Subsystem9 ==
  u : Inport
  w : Inport  Port=2
  Gain : Gain  Gain=A  Multiplication=Matrix(K*u)
  Gain1 : Gain  Gain=B  Multiplication=Matrix(K*u)
  Gain2 : Gain  Gain=E  Multiplication=Matrix(K*u)
  Gain3 : Gain  Gain=C  Multiplication=Matrix(K*u)
  Gain4 : Gain  Gain=D  Multiplication=Matrix(K*u)
  Gain5 : Gain  Gain=F  Multiplication=Matrix(K*u)
  Gain6 : Gain  Gain=G  Multiplication=Matrix(K*u)
  Gain7 : Gain  Gain=H  Multiplication=Matrix(K*u)
  Gain8 : Gain  Gain=J  Multiplication=Matrix(K*u)
  Integrator : Integrator  InitialCondition=10*ones(n,1)
  Sum : Sum  Inputs=+++
  Sum1 : Sum  Inputs=+++
  Sum2 : Sum  Inputs=+++
  y : Outport
  z : Outport  Port=2
  x : Outport  Port=3
  wires:
  u/1 -> Gain7/1, Gain4/1, Gain1/1  "u"
  Gain2/1 -> Sum/3
  w/1 -> Gain8/1, Gain5/1, Gain2/1  "w"
  Gain3/1 -> Sum1/1
  Sum/1 -> Integrator/1  "xDot"
  Gain5/1 -> Sum1/3
  Gain/1 -> Sum/1
  Gain1/1 -> Sum/2
  Integrator/1 -> x/1, Gain6/1, Gain3/1, Gain/1  "x"
  Gain4/1 -> Sum1/2
  Sum2/1 -> z/1  "z"
  Sum1/1 -> y/1  "y"
  Gain8/1 -> Sum2/3
  Gain6/1 -> Sum2/1
  Gain7/1 -> Sum2/2
